simulink model "RAM_Design"  (R2025a)
settings: Solver=FixedStepDiscrete  StartTime=0.0  StopTime=10  FixedStep=1e-6  RelTol=1e-3
undefined symbols (not defined in the file): Bit_1, Bit_2, Bit_3, Bit_4, Bit_5, Bit_6, Bit_7, Bit_8
libraries: fl_lib x320, nesl_utility x136, simulink_extras x57
(part 5 of 5)

== system RAM_Design/Subsystem1/8Bit RAM 8/Subsystem16/Subsystem4 ==
  Cast To Boolean : DataTypeConversion  OutDataTypeStr=boolean  SaturateOnIntegerOverflow=off  RndMeth=Floor
  Delay One Step : Delay  DelayLength=1
  Electrical Reference : fl_lib/Electrical/Electrical Elements/Electrical Reference
  Gain : Gain  Gain=0.2
  PS-Simulink Converter : nesl_utility/PS-Simulink Converter  PhysicalDomain=network_engine_domain  SubClassName=ps_output  LeftPortType=input  RightPortType=output  PseudoPeriodic=off  Frequencies=[]  VectorFormat=inherit  Unit=inherit  AffineConversion=off
  Voltage Sensor : fl_lib/Electrical/Electrical Sensors/Voltage Sensor
  PS : PMIOPort  Side=Left
  SIM : Outport
  wires:
  PS-Simulink Converter/1 -> Gain/1
  Cast To Boolean/1 -> Delay One Step/1
  Gain/1 -> Cast To Boolean/1
  Delay One Step/1 -> SIM/1
  connections:
  PS/RConn1 -- Voltage Sensor/LConn1
  Electrical Reference/LConn1 -- Voltage Sensor/RConn2
  PS-Simulink Converter/LConn1 -- Voltage Sensor/RConn1

== system RAM_Design/Subsystem1/8Bit RAM 8/Subsystem16/Subsystem5 ==
  Cast To Boolean : DataTypeConversion  OutDataTypeStr=boolean  SaturateOnIntegerOverflow=off  RndMeth=Floor
  Delay One Step : Delay  DelayLength=1
  Electrical Reference : fl_lib/Electrical/Electrical Elements/Electrical Reference
  Gain : Gain  Gain=0.2
  PS-Simulink Converter : nesl_utility/PS-Simulink Converter  PhysicalDomain=network_engine_domain  SubClassName=ps_output  LeftPortType=input  RightPortType=output  PseudoPeriodic=off  Frequencies=[]  VectorFormat=inherit  Unit=inherit  AffineConversion=off
  Voltage Sensor : fl_lib/Electrical/Electrical Sensors/Voltage Sensor
  PS : PMIOPort  Side=Left
  SIM : Outport
  wires:
  PS-Simulink Converter/1 -> Gain/1
  Cast To Boolean/1 -> Delay One Step/1
  Gain/1 -> Cast To Boolean/1
  Delay One Step/1 -> SIM/1
  connections:
  PS/RConn1 -- Voltage Sensor/LConn1
  Electrical Reference/LConn1 -- Voltage Sensor/RConn2
  PS-Simulink Converter/LConn1 -- Voltage Sensor/RConn1

== system RAM_Design/Subsystem1/8Bit RAM 8/Subsystem16/Subsystem6 ==
  Cast To Boolean : DataTypeConversion  OutDataTypeStr=boolean  SaturateOnIntegerOverflow=off  RndMeth=Floor
  Delay One Step : Delay  DelayLength=1
  Electrical Reference : fl_lib/Electrical/Electrical Elements/Electrical Reference
  Gain : Gain  Gain=0.2
  PS-Simulink Converter : nesl_utility/PS-Simulink Converter  PhysicalDomain=network_engine_domain  SubClassName=ps_output  LeftPortType=input  RightPortType=output  PseudoPeriodic=off  Frequencies=[]  VectorFormat=inherit  Unit=inherit  AffineConversion=off
  Voltage Sensor : fl_lib/Electrical/Electrical Sensors/Voltage Sensor
  PS : PMIOPort  Side=Left
  SIM : Outport
  wires:
  PS-Simulink Converter/1 -> Gain/1
  Cast To Boolean/1 -> Delay One Step/1
  Gain/1 -> Cast To Boolean/1
  Delay One Step/1 -> SIM/1
  connections:
  PS/RConn1 -- Voltage Sensor/LConn1
  Electrical Reference/LConn1 -- Voltage Sensor/RConn2
  PS-Simulink Converter/LConn1 -- Voltage Sensor/RConn1

== system RAM_Design/Subsystem1/8Bit RAM 8/Subsystem16/Subsystem7 ==
  Cast To Boolean : DataTypeConversion  OutDataTypeStr=boolean  SaturateOnIntegerOverflow=off  RndMeth=Floor
  Delay One Step : Delay  DelayLength=1
  Electrical Reference : fl_lib/Electrical/Electrical Elements/Electrical Reference
  Gain : Gain  Gain=0.2
  PS-Simulink Converter : nesl_utility/PS-Simulink Converter  PhysicalDomain=network_engine_domain  SubClassName=ps_output  LeftPortType=input  RightPortType=output  PseudoPeriodic=off  Frequencies=[]  VectorFormat=inherit  Unit=inherit  AffineConversion=off
  Voltage Sensor : fl_lib/Electrical/Electrical Sensors/Voltage Sensor
  PS : PMIOPort  Side=Left
  SIM : Outport
  wires:
  PS-Simulink Converter/1 -> Gain/1
  Cast To Boolean/1 -> Delay One Step/1
  Gain/1 -> Cast To Boolean/1
  Delay One Step/1 -> SIM/1
  connections:
  PS/RConn1 -- Voltage Sensor/LConn1
  Electrical Reference/LConn1 -- Voltage Sensor/RConn2
  PS-Simulink Converter/LConn1 -- Voltage Sensor/RConn1

== system RAM_Design/Subsystem1/8Bit RAM 8/Subsystem16/Subsystem8 ==
  Cast To Boolean : DataTypeConversion  OutDataTypeStr=boolean  SaturateOnIntegerOverflow=off  RndMeth=Floor
  Delay One Step : Delay  DelayLength=1
  Electrical Reference : fl_lib/Electrical/Electrical Elements/Electrical Reference
  Gain : Gain  Gain=0.2
  PS-Simulink Converter : nesl_utility/PS-Simulink Converter  PhysicalDomain=network_engine_domain  SubClassName=ps_output  LeftPortType=input  RightPortType=output  PseudoPeriodic=off  Frequencies=[]  VectorFormat=inherit  Unit=inherit  AffineConversion=off
  Voltage Sensor : fl_lib/Electrical/Electrical Sensors/Voltage Sensor
  PS : PMIOPort  Side=Left
  SIM : Outport
  wires:
  PS-Simulink Converter/1 -> Gain/1
  Cast To Boolean/1 -> Delay One Step/1
  Gain/1 -> Cast To Boolean/1
  Delay One Step/1 -> SIM/1
  connections:
  PS/RConn1 -- Voltage Sensor/LConn1
  Electrical Reference/LConn1 -- Voltage Sensor/RConn2
  PS-Simulink Converter/LConn1 -- Voltage Sensor/RConn1

== matlab function RAM_Design/MATLAB Function ==
  data: StoreMar output; CLK input; Read output; Write output; Databus output
function [StoreMar,Read,Write,Databus]= fcn(CLK)
